simulink model "active_vehicle_ESP_Control"  (R2020a)
settings: Solver=ode4  StartTime=0.0  StopTime=inf  FixedStep=1e-3  RelTol=1e-3
InitFcn:
  | clear mex
model workspace (MAT data in the model file):
  inChnlList : object (value not decoded)
  inChnlListInternal : object (value not decoded)
  outChnlList : object (value not decoded)
  outChnlListInternal : object (value not decoded)
undefined symbols (not defined in the file or in its folder): DiscIntNeverNeededParam, vicrt_initcallback, vicrt_initmexcallback, vicrt_inputfile, vicrt_simulationmanager
libraries: simulink x1
(part 6 of 6)

== system active_vehicle_ESP_Control/Vehicle/VI-CarRealTime/Input_Bus/Inputs/Irregularity/road ==
  BCroad : BusCreator  Inputs=4
  L1_def_val : Constant  Value=0
  L2_def_val : Constant  Value=0
  R1_def_val : Constant  Value=0
  R2_def_val : Constant  Value=0
  road : Outport
  wires:
  BCroad/1 -> road/1  "road"
  L1_def_val/1 -> BCroad/1  "L1"
  L2_def_val/1 -> BCroad/2  "L2"
  R1_def_val/1 -> BCroad/3  "R1"
  R2_def_val/1 -> BCroad/4  "R2"

== system active_vehicle_ESP_Control/Vehicle/VI-CarRealTime/Input_Bus/Inputs/Main_Bumpstop/activity_flag ==
  BCactivity_flag : BusCreator  Inputs=4
  L1_def_val : Constant
  L2_def_val : Constant
  R1_def_val : Constant
  R2_def_val : Constant
  activity_flag : Outport
  wires:
  BCactivity_flag/1 -> activity_flag/1  "activity_flag"
  L1_def_val/1 -> BCactivity_flag/1  "L1"
  L2_def_val/1 -> BCactivity_flag/2  "L2"
  R1_def_val/1 -> BCactivity_flag/3  "R1"
  R2_def_val/1 -> BCactivity_flag/4  "R2"

== system active_vehicle_ESP_Control/Vehicle/VI-CarRealTime/Input_Bus/Inputs/Main_Bumpstop/force ==
  BCforce : BusCreator  Inputs=4
  L1_def_val : Constant  Value=0
  L2_def_val : Constant  Value=0
  R1_def_val : Constant  Value=0
  R2_def_val : Constant  Value=0
  force : Outport
  wires:
  BCforce/1 -> force/1  "force"
  L1_def_val/1 -> BCforce/1  "L1"
  L2_def_val/1 -> BCforce/2  "L2"
  R1_def_val/1 -> BCforce/3  "R1"
  R2_def_val/1 -> BCforce/4  "R2"

== system active_vehicle_ESP_Control/Vehicle/VI-CarRealTime/Input_Bus/Inputs/Main_Damper/activity_flag ==
  BCactivity_flag : BusCreator  Inputs=4
  L1_def_val : Constant
  L2_def_val : Constant
  R1_def_val : Constant
  R2_def_val : Constant
  activity_flag : Outport
  wires:
  BCactivity_flag/1 -> activity_flag/1  "activity_flag"
  L1_def_val/1 -> BCactivity_flag/1  "L1"
  L2_def_val/1 -> BCactivity_flag/2  "L2"
  R1_def_val/1 -> BCactivity_flag/3  "R1"
  R2_def_val/1 -> BCactivity_flag/4  "R2"

== system active_vehicle_ESP_Control/Vehicle/VI-CarRealTime/Input_Bus/Inputs/Main_Damper/force ==
  BCforce : BusCreator  Inputs=4
  L1_def_val : Constant  Value=0
  L2_def_val : Constant  Value=0
  R1_def_val : Constant  Value=0
  R2_def_val : Constant  Value=0
  force : Outport
  wires:
  BCforce/1 -> force/1  "force"
  L1_def_val/1 -> BCforce/1  "L1"
  L2_def_val/1 -> BCforce/2  "L2"
  R1_def_val/1 -> BCforce/3  "R1"
  R2_def_val/1 -> BCforce/4  "R2"

== system active_vehicle_ESP_Control/Vehicle/VI-CarRealTime/Input_Bus/Inputs/Main_Inerter/activity_flag ==
  BCactivity_flag : BusCreator  Inputs=4
  L1_def_val : Constant
  L2_def_val : Constant
  R1_def_val : Constant
  R2_def_val : Constant
  activity_flag : Outport
  wires:
  BCactivity_flag/1 -> activity_flag/1  "activity_flag"
  L1_def_val/1 -> BCactivity_flag/1  "L1"
  L2_def_val/1 -> BCactivity_flag/2  "L2"
  R1_def_val/1 -> BCactivity_flag/3  "R1"
  R2_def_val/1 -> BCactivity_flag/4  "R2"

== system active_vehicle_ESP_Control/Vehicle/VI-CarRealTime/Input_Bus/Inputs/Main_Inerter/force ==
  BCforce : BusCreator  Inputs=4
  L1_def_val : Constant  Value=0
  L2_def_val : Constant  Value=0
  R1_def_val : Constant  Value=0
  R2_def_val : Constant  Value=0
  force : Outport
  wires:
  BCforce/1 -> force/1  "force"
  L1_def_val/1 -> BCforce/1  "L1"
  L2_def_val/1 -> BCforce/2  "L2"
  R1_def_val/1 -> BCforce/3  "R1"
  R2_def_val/1 -> BCforce/4  "R2"

== system active_vehicle_ESP_Control/Vehicle/VI-CarRealTime/Input_Bus/Inputs/Main_Reboundstop/activity_flag ==
  BCactivity_flag : BusCreator  Inputs=4
  L1_def_val : Constant
  L2_def_val : Constant
  R1_def_val : Constant
  R2_def_val : Constant
  activity_flag : Outport
  wires:
  BCactivity_flag/1 -> activity_flag/1  "activity_flag"
  L1_def_val/1 -> BCactivity_flag/1  "L1"
  L2_def_val/1 -> BCactivity_flag/2  "L2"
  R1_def_val/1 -> BCactivity_flag/3  "R1"
  R2_def_val/1 -> BCactivity_flag/4  "R2"

== system active_vehicle_ESP_Control/Vehicle/VI-CarRealTime/Input_Bus/Inputs/Main_Reboundstop/force ==
  BCforce : BusCreator  Inputs=4
  L1_def_val : Constant  Value=0
  L2_def_val : Constant  Value=0
  R1_def_val : Constant  Value=0
  R2_def_val : Constant  Value=0
  force : Outport
  wires:
  BCforce/1 -> force/1  "force"
  L1_def_val/1 -> BCforce/1  "L1"
  L2_def_val/1 -> BCforce/2  "L2"
  R1_def_val/1 -> BCforce/3  "R1"
  R2_def_val/1 -> BCforce/4  "R2"

== system active_vehicle_ESP_Control/Vehicle/VI-CarRealTime/Input_Bus/Inputs/Main_Spring/activity_flag ==
  BCactivity_flag : BusCreator  Inputs=4
  L1_def_val : Constant
  L2_def_val : Constant
  R1_def_val : Constant
  R2_def_val : Constant
  activity_flag : Outport
  wires:
  BCactivity_flag/1 -> activity_flag/1  "activity_flag"
  L1_def_val/1 -> BCactivity_flag/1  "L1"
  L2_def_val/1 -> BCactivity_flag/2  "L2"
  R1_def_val/1 -> BCactivity_flag/3  "R1"
  R2_def_val/1 -> BCactivity_flag/4  "R2"

== system active_vehicle_ESP_Control/Vehicle/VI-CarRealTime/Input_Bus/Inputs/Main_Spring/force ==
  BCforce : BusCreator  Inputs=4
  L1_def_val : Constant  Value=0
  L2_def_val : Constant  Value=0
  R1_def_val : Constant  Value=0
  R2_def_val : Constant  Value=0
  force : Outport
  wires:
  BCforce/1 -> force/1  "force"
  L1_def_val/1 -> BCforce/1  "L1"
  L2_def_val/1 -> BCforce/2  "L2"
  R1_def_val/1 -> BCforce/3  "R1"
  R2_def_val/1 -> BCforce/4  "R2"

== system active_vehicle_ESP_Control/Vehicle/VI-CarRealTime/Input_Bus/Inputs/Mono_Element/Bumpstop_Damper ==
  BCBumpstop_Damper : BusCreator  Inputs=2
  front_def_val : Constant  Value=0
  rear_def_val : Constant  Value=0
  Bumpstop_Damper : Outport
  wires:
  BCBumpstop_Damper/1 -> Bumpstop_Damper/1  "Bumpstop_Damper"
  front_def_val/1 -> BCBumpstop_Damper/1  "front"
  rear_def_val/1 -> BCBumpstop_Damper/2  "rear"

== system active_vehicle_ESP_Control/Vehicle/VI-CarRealTime/Input_Bus/Inputs/Mono_Element/Bumpstop_Damper_activity_flag ==
  BCBumpstop_Damper_activity_flag : BusCreator  Inputs=2
  front_def_val : Constant
  rear_def_val : Constant
  Bumpstop_Damper_activity_flag : Outport
  wires:
  BCBumpstop_Damper_activity_flag/1 -> Bumpstop_Damper_activity_flag/1  "Bumpstop_Damper_activity_flag"
  front_def_val/1 -> BCBumpstop_Damper_activity_flag/1  "front"
  rear_def_val/1 -> BCBumpstop_Damper_activity_flag/2  "rear"

== system active_vehicle_ESP_Control/Vehicle/VI-CarRealTime/Input_Bus/Inputs/Mono_Element/Bumpstop_Spring ==
  BCBumpstop_Spring : BusCreator  Inputs=2
  front_def_val : Constant  Value=0
  rear_def_val : Constant  Value=0
  Bumpstop_Spring : Outport
  wires:
  BCBumpstop_Spring/1 -> Bumpstop_Spring/1  "Bumpstop_Spring"
  front_def_val/1 -> BCBumpstop_Spring/1  "front"
  rear_def_val/1 -> BCBumpstop_Spring/2  "rear"

== system active_vehicle_ESP_Control/Vehicle/VI-CarRealTime/Input_Bus/Inputs/Mono_Element/Bumpstop_Spring_activity_flag ==
  BCBumpstop_Spring_activity_flag : BusCreator  Inputs=2
  front_def_val : Constant
  rear_def_val : Constant
  Bumpstop_Spring_activity_flag : Outport
  wires:
  BCBumpstop_Spring_activity_flag/1 -> Bumpstop_Spring_activity_flag/1  "Bumpstop_Spring_activity_flag"
  front_def_val/1 -> BCBumpstop_Spring_activity_flag/1  "front"
  rear_def_val/1 -> BCBumpstop_Spring_activity_flag/2  "rear"

== system active_vehicle_ESP_Control/Vehicle/VI-CarRealTime/Input_Bus/Inputs/Mono_Element/Damper ==
  BCDamper : BusCreator  Inputs=2
  front_def_val : Constant  Value=0
  rear_def_val : Constant  Value=0
  Damper : Outport
  wires:
  BCDamper/1 -> Damper/1  "Damper"
  front_def_val/1 -> BCDamper/1  "front"
  rear_def_val/1 -> BCDamper/2  "rear"

== system active_vehicle_ESP_Control/Vehicle/VI-CarRealTime/Input_Bus/Inputs/Mono_Element/Damper_activity_flag ==
  BCDamper_activity_flag : BusCreator  Inputs=2
  front_def_val : Constant
  rear_def_val : Constant
  Damper_activity_flag : Outport
  wires:
  BCDamper_activity_flag/1 -> Damper_activity_flag/1  "Damper_activity_flag"
  front_def_val/1 -> BCDamper_activity_flag/1  "front"
  rear_def_val/1 -> BCDamper_activity_flag/2  "rear"

== system active_vehicle_ESP_Control/Vehicle/VI-CarRealTime/Input_Bus/Inputs/Mono_Element/Inerter ==
  BCInerter : BusCreator  Inputs=2
  front_def_val : Constant  Value=0
  rear_def_val : Constant  Value=0
  Inerter : Outport
  wires:
  BCInerter/1 -> Inerter/1  "Inerter"
  front_def_val/1 -> BCInerter/1  "front"
  rear_def_val/1 -> BCInerter/2  "rear"

== system active_vehicle_ESP_Control/Vehicle/VI-CarRealTime/Input_Bus/Inputs/Mono_Element/Inerter_activity_flag ==
  BCInerter_activity_flag : BusCreator  Inputs=2
  front_def_val : Constant
  rear_def_val : Constant
  Inerter_activity_flag : Outport
  wires:
  BCInerter_activity_flag/1 -> Inerter_activity_flag/1  "Inerter_activity_flag"
  front_def_val/1 -> BCInerter_activity_flag/1  "front"
  rear_def_val/1 -> BCInerter_activity_flag/2  "rear"

== system active_vehicle_ESP_Control/Vehicle/VI-CarRealTime/Input_Bus/Inputs/Mono_Element/Reboundstop_Damper ==
  BCReboundstop_Damper : BusCreator  Inputs=2
  front_def_val : Constant  Value=0
  rear_def_val : Constant  Value=0
  Reboundstop_Damper : Outport
  wires:
  BCReboundstop_Damper/1 -> Reboundstop_Damper/1  "Reboundstop_Damper"
  front_def_val/1 -> BCReboundstop_Damper/1  "front"
  rear_def_val/1 -> BCReboundstop_Damper/2  "rear"

== system active_vehicle_ESP_Control/Vehicle/VI-CarRealTime/Input_Bus/Inputs/Mono_Element/Reboundstop_Damper_activity_flag ==
  BCReboundstop_Damper_activity_flag : BusCreator  Inputs=2
  front_def_val : Constant
  rear_def_val : Constant
  Reboundstop_Damper_activity_flag : Outport
  wires:
  BCReboundstop_Damper_activity_flag/1 -> Reboundstop_Damper_activity_flag/1  "Reboundstop_Damper_activity_flag"
  front_def_val/1 -> BCReboundstop_Damper_activity_flag/1  "front"
  rear_def_val/1 -> BCReboundstop_Damper_activity_flag/2  "rear"

== system active_vehicle_ESP_Control/Vehicle/VI-CarRealTime/Input_Bus/Inputs/Mono_Element/Reboundstop_Spring ==
  BCReboundstop_Spring : BusCreator  Inputs=2
  front_def_val : Constant  Value=0
  rear_def_val : Constant  Value=0
  Reboundstop_Spring : Outport
  wires:
  BCReboundstop_Spring/1 -> Reboundstop_Spring/1  "Reboundstop_Spring"
  front_def_val/1 -> BCReboundstop_Spring/1  "front"
  rear_def_val/1 -> BCReboundstop_Spring/2  "rear"

== system active_vehicle_ESP_Control/Vehicle/VI-CarRealTime/Input_Bus/Inputs/Mono_Element/Reboundstop_Spring_activity_flag ==
  BCReboundstop_Spring_activity_flag : BusCreator  Inputs=2
  front_def_val : Constant
  rear_def_val : Constant
  Reboundstop_Spring_activity_flag : Outport
  wires:
  BCReboundstop_Spring_activity_flag/1 -> Reboundstop_Spring_activity_flag/1  "Reboundstop_Spring_activity_flag"
  front_def_val/1 -> BCReboundstop_Spring_activity_flag/1  "front"
  rear_def_val/1 -> BCReboundstop_Spring_activity_flag/2  "rear"

== system active_vehicle_ESP_Control/Vehicle/VI-CarRealTime/Input_Bus/Inputs/Mono_Element/Roll_Damper ==
  BCRoll_Damper : BusCreator  Inputs=2
  front_def_val : Constant  Value=0
  rear_def_val : Constant  Value=0
  Roll_Damper : Outport
  wires:
  BCRoll_Damper/1 -> Roll_Damper/1  "Roll_Damper"
  front_def_val/1 -> BCRoll_Damper/1  "front"
  rear_def_val/1 -> BCRoll_Damper/2  "rear"

== system active_vehicle_ESP_Control/Vehicle/VI-CarRealTime/Input_Bus/Inputs/Mono_Element/Roll_Damper_activity_flag ==
  BCRoll_Damper_activity_flag : BusCreator  Inputs=2
  front_def_val : Constant
  rear_def_val : Constant
  Roll_Damper_activity_flag : Outport
  wires:
  BCRoll_Damper_activity_flag/1 -> Roll_Damper_activity_flag/1  "Roll_Damper_activity_flag"
  front_def_val/1 -> BCRoll_Damper_activity_flag/1  "front"
  rear_def_val/1 -> BCRoll_Damper_activity_flag/2  "rear"

== system active_vehicle_ESP_Control/Vehicle/VI-CarRealTime/Input_Bus/Inputs/Mono_Element/Spring ==
  BCSpring : BusCreator  Inputs=2
  front_def_val : Constant  Value=0
  rear_def_val : Constant  Value=0
  Spring : Outport
  wires:
  BCSpring/1 -> Spring/1  "Spring"
  front_def_val/1 -> BCSpring/1  "front"
  rear_def_val/1 -> BCSpring/2  "rear"

== system active_vehicle_ESP_Control/Vehicle/VI-CarRealTime/Input_Bus/Inputs/Mono_Element/Spring_activity_flag ==
  BCSpring_activity_flag : BusCreator  Inputs=2
  front_def_val : Constant
  rear_def_val : Constant
  Spring_activity_flag : Outport
  wires:
  BCSpring_activity_flag/1 -> Spring_activity_flag/1  "Spring_activity_flag"
  front_def_val/1 -> BCSpring_activity_flag/1  "front"
  rear_def_val/1 -> BCSpring_activity_flag/2  "rear"

== system active_vehicle_ESP_Control/Vehicle/VI-CarRealTime/Input_Bus/Inputs/Rear_Steering_Actuator_disp/str_swa ==
  BCstr_swa : BusCreator  Inputs=2
  left_def_val : Constant  Value=0
  right_def_val : Constant  Value=0
  str_swa : Outport
  wires:
  BCstr_swa/1 -> str_swa/1  "str_swa"
  left_def_val/1 -> BCstr_swa/1  "left"
  right_def_val/1 -> BCstr_swa/2  "right"

== system active_vehicle_ESP_Control/Vehicle/VI-CarRealTime/Input_Bus/Inputs/Steering/steer_at_spindle ==
  BCsteer_at_spindle : BusCreator  Inputs=4
  L1_def_val : Constant  Value=0
  L2_def_val : Constant  Value=0
  R1_def_val : Constant  Value=0
  R2_def_val : Constant  Value=0
  steer_at_spindle : Outport
  wires:
  BCsteer_at_spindle/1 -> steer_at_spindle/1  "steer_at_spindle"
  L1_def_val/1 -> BCsteer_at_spindle/1  "L1"
  L2_def_val/1 -> BCsteer_at_spindle/2  "L2"
  R1_def_val/1 -> BCsteer_at_spindle/3  "R1"
  R2_def_val/1 -> BCsteer_at_spindle/4  "R2"

== system active_vehicle_ESP_Control/Vehicle/VI-CarRealTime/Input_Bus/Inputs/Subsystem_Activation/Internal_Brake_System_Activity ==
  BCInternal_Brake_System_Activity : BusCreator  Inputs=4
  L1_def_val : Constant
  L2_def_val : Constant
  R1_def_val : Constant
  R2_def_val : Constant
  Internal_Brake_System_Activity : Outport
  wires:
  BCInternal_Brake_System_Activity/1 -> Internal_Brake_System_Activity/1  "Internal_Brake_System_Activity"
  L1_def_val/1 -> BCInternal_Brake_System_Activity/1  "L1"
  L2_def_val/1 -> BCInternal_Brake_System_Activity/2  "L2"
  R1_def_val/1 -> BCInternal_Brake_System_Activity/3  "R1"
  R2_def_val/1 -> BCInternal_Brake_System_Activity/4  "R2"

== system active_vehicle_ESP_Control/Vehicle/VI-CarRealTime/Input_Bus/Inputs/Subsystem_Activation/Tire_Force_x ==
  BCTire_Force_x : BusCreator  Inputs=4
  L1_def_val : Constant
  L2_def_val : Constant
  R1_def_val : Constant
  R2_def_val : Constant
  Tire_Force_x : Outport
  wires:
  BCTire_Force_x/1 -> Tire_Force_x/1  "Tire_Force_x"
  L1_def_val/1 -> BCTire_Force_x/1  "L1"
  L2_def_val/1 -> BCTire_Force_x/2  "L2"
  R1_def_val/1 -> BCTire_Force_x/3  "R1"
  R2_def_val/1 -> BCTire_Force_x/4  "R2"

== system active_vehicle_ESP_Control/Vehicle/VI-CarRealTime/Input_Bus/Inputs/Subsystem_Activation/Tire_Force_y ==
  BCTire_Force_y : BusCreator  Inputs=4
  L1_def_val : Constant
  L2_def_val : Constant
  R1_def_val : Constant
  R2_def_val : Constant
  Tire_Force_y : Outport
  wires:
  BCTire_Force_y/1 -> Tire_Force_y/1  "Tire_Force_y"
  L1_def_val/1 -> BCTire_Force_y/1  "L1"
  L2_def_val/1 -> BCTire_Force_y/2  "L2"
  R1_def_val/1 -> BCTire_Force_y/3  "R1"
  R2_def_val/1 -> BCTire_Force_y/4  "R2"

== system active_vehicle_ESP_Control/Vehicle/VI-CarRealTime/Input_Bus/Inputs/Subsystem_Activation/Tire_Force_z ==
  BCTire_Force_z : BusCreator  Inputs=4
  L1_def_val : Constant
  L2_def_val : Constant
  R1_def_val : Constant
  R2_def_val : Constant
  Tire_Force_z : Outport
  wires:
  BCTire_Force_z/1 -> Tire_Force_z/1  "Tire_Force_z"
  L1_def_val/1 -> BCTire_Force_z/1  "L1"
  L2_def_val/1 -> BCTire_Force_z/2  "L2"
  R1_def_val/1 -> BCTire_Force_z/3  "R1"
  R2_def_val/1 -> BCTire_Force_z/4  "R2"

== system active_vehicle_ESP_Control/Vehicle/VI-CarRealTime/Input_Bus/Inputs/Subsystem_Activation/Tire_Moment_x ==
  BCTire_Moment_x : BusCreator  Inputs=4
  L1_def_val : Constant
  L2_def_val : Constant
  R1_def_val : Constant
  R2_def_val : Constant
  Tire_Moment_x : Outport
  wires:
  BCTire_Moment_x/1 -> Tire_Moment_x/1  "Tire_Moment_x"
  L1_def_val/1 -> BCTire_Moment_x/1  "L1"
  L2_def_val/1 -> BCTire_Moment_x/2  "L2"
  R1_def_val/1 -> BCTire_Moment_x/3  "R1"
  R2_def_val/1 -> BCTire_Moment_x/4  "R2"

== system active_vehicle_ESP_Control/Vehicle/VI-CarRealTime/Input_Bus/Inputs/Subsystem_Activation/Tire_Moment_y ==
  BCTire_Moment_y : BusCreator  Inputs=4
  L1_def_val : Constant
  L2_def_val : Constant
  R1_def_val : Constant
  R2_def_val : Constant
  Tire_Moment_y : Outport
  wires:
  BCTire_Moment_y/1 -> Tire_Moment_y/1  "Tire_Moment_y"
  L1_def_val/1 -> BCTire_Moment_y/1  "L1"
  L2_def_val/1 -> BCTire_Moment_y/2  "L2"
  R1_def_val/1 -> BCTire_Moment_y/3  "R1"
  R2_def_val/1 -> BCTire_Moment_y/4  "R2"

== system active_vehicle_ESP_Control/Vehicle/VI-CarRealTime/Input_Bus/Inputs/Subsystem_Activation/Tire_Moment_z ==
  BCTire_Moment_z : BusCreator  Inputs=4
  L1_def_val : Constant
  L2_def_val : Constant
  R1_def_val : Constant
  R2_def_val : Constant
  Tire_Moment_z : Outport
  wires:
  BCTire_Moment_z/1 -> Tire_Moment_z/1  "Tire_Moment_z"
  L1_def_val/1 -> BCTire_Moment_z/1  "L1"
  L2_def_val/1 -> BCTire_Moment_z/2  "L2"
  R1_def_val/1 -> BCTire_Moment_z/3  "R1"
  R2_def_val/1 -> BCTire_Moment_z/4  "R2"

== system active_vehicle_ESP_Control/Vehicle/VI-CarRealTime/Input_Bus/Inputs/Third_Element/Damper_activity_flag ==
  BCDamper_activity_flag : BusCreator  Inputs=2
  front_def_val : Constant
  rear_def_val : Constant
  Damper_activity_flag : Outport
  wires:
  BCDamper_activity_flag/1 -> Damper_activity_flag/1  "Damper_activity_flag"
  front_def_val/1 -> BCDamper_activity_flag/1  "front"
  rear_def_val/1 -> BCDamper_activity_flag/2  "rear"

== system active_vehicle_ESP_Control/Vehicle/VI-CarRealTime/Input_Bus/Inputs/Third_Element/Damper_force ==
  BCDamper_force : BusCreator  Inputs=2
  front_def_val : Constant  Value=0
  rear_def_val : Constant  Value=0
  Damper_force : Outport
  wires:
  BCDamper_force/1 -> Damper_force/1  "Damper_force"
  front_def_val/1 -> BCDamper_force/1  "front"
  rear_def_val/1 -> BCDamper_force/2  "rear"

== system active_vehicle_ESP_Control/Vehicle/VI-CarRealTime/Input_Bus/Inputs/Third_Element/Spring ==
  BCSpring : BusCreator  Inputs=2
  front_def_val : Constant  Value=0
  rear_def_val : Constant  Value=0
  Spring : Outport
  wires:
  BCSpring/1 -> Spring/1  "Spring"
  front_def_val/1 -> BCSpring/1  "front"
  rear_def_val/1 -> BCSpring/2  "rear"

== system active_vehicle_ESP_Control/Vehicle/VI-CarRealTime/Input_Bus/Inputs/Third_Element/Spring_activity_flag ==
  BCSpring_activity_flag : BusCreator  Inputs=2
  front_def_val : Constant
  rear_def_val : Constant
  Spring_activity_flag : Outport
  wires:
  BCSpring_activity_flag/1 -> Spring_activity_flag/1  "Spring_activity_flag"
  front_def_val/1 -> BCSpring_activity_flag/1  "front"
  rear_def_val/1 -> BCSpring_activity_flag/2  "rear"

== system active_vehicle_ESP_Control/Vehicle/VI-CarRealTime/Input_Bus/Inputs/Tire_Force/Fx ==
  BCFx : BusCreator  Inputs=4
  L1_def_val : Constant  Value=0
  L2_def_val : Constant  Value=0
  R1_def_val : Constant  Value=0
  R2_def_val : Constant  Value=0
  Fx : Outport
  wires:
  BCFx/1 -> Fx/1  "Fx"
  L1_def_val/1 -> BCFx/1  "L1"
  L2_def_val/1 -> BCFx/2  "L2"
  R1_def_val/1 -> BCFx/3  "R1"
  R2_def_val/1 -> BCFx/4  "R2"

== system active_vehicle_ESP_Control/Vehicle/VI-CarRealTime/Input_Bus/Inputs/Tire_Force/Fy ==
  BCFy : BusCreator  Inputs=4
  L1_def_val : Constant  Value=0
  L2_def_val : Constant  Value=0
  R1_def_val : Constant  Value=0
  R2_def_val : Constant  Value=0
  Fy : Outport
  wires:
  BCFy/1 -> Fy/1  "Fy"
  L1_def_val/1 -> BCFy/1  "L1"
  L2_def_val/1 -> BCFy/2  "L2"
  R1_def_val/1 -> BCFy/3  "R1"
  R2_def_val/1 -> BCFy/4  "R2"

== system active_vehicle_ESP_Control/Vehicle/VI-CarRealTime/Input_Bus/Inputs/Tire_Force/Fz ==
  BCFz : BusCreator  Inputs=4
  L1_def_val : Constant  Value=0
  L2_def_val : Constant  Value=0
  R1_def_val : Constant  Value=0
  R2_def_val : Constant  Value=0
  Fz : Outport
  wires:
  BCFz/1 -> Fz/1  "Fz"
  L1_def_val/1 -> BCFz/1  "L1"
  L2_def_val/1 -> BCFz/2  "L2"
  R1_def_val/1 -> BCFz/3  "R1"
  R2_def_val/1 -> BCFz/4  "R2"

== system active_vehicle_ESP_Control/Vehicle/VI-CarRealTime/Input_Bus/Inputs/Tire_Moment/Mx ==
  BCMx : BusCreator  Inputs=4
  L1_def_val : Constant  Value=0
  L2_def_val : Constant  Value=0
  R1_def_val : Constant  Value=0
  R2_def_val : Constant  Value=0
  Mx : Outport
  wires:
  BCMx/1 -> Mx/1  "Mx"
  L1_def_val/1 -> BCMx/1  "L1"
  L2_def_val/1 -> BCMx/2  "L2"
  R1_def_val/1 -> BCMx/3  "R1"
  R2_def_val/1 -> BCMx/4  "R2"

== system active_vehicle_ESP_Control/Vehicle/VI-CarRealTime/Input_Bus/Inputs/Tire_Moment/My ==
  BCMy : BusCreator  Inputs=4
  L1_def_val : Constant  Value=0
  L2_def_val : Constant  Value=0
  R1_def_val : Constant  Value=0
  R2_def_val : Constant  Value=0
  My : Outport
  wires:
  BCMy/1 -> My/1  "My"
  L1_def_val/1 -> BCMy/1  "L1"
  L2_def_val/1 -> BCMy/2  "L2"
  R1_def_val/1 -> BCMy/3  "R1"
  R2_def_val/1 -> BCMy/4  "R2"

== system active_vehicle_ESP_Control/Vehicle/VI-CarRealTime/Input_Bus/Inputs/Tire_Moment/Mz ==
  BCMz : BusCreator  Inputs=4
  L1_def_val : Constant  Value=0
  L2_def_val : Constant  Value=0
  R1_def_val : Constant  Value=0
  R2_def_val : Constant  Value=0
  Mz : Outport
  wires:
  BCMz/1 -> Mz/1  "Mz"
  L1_def_val/1 -> BCMz/1  "L1"
  L2_def_val/1 -> BCMz/2  "L2"
  R1_def_val/1 -> BCMz/3  "R1"
  R2_def_val/1 -> BCMz/4  "R2"

== system active_vehicle_ESP_Control/Vehicle/VI-CarRealTime/Input_Bus/Inputs/Wheel_driving/moment ==
  BCmoment : BusCreator  Inputs=4
  L1_def_val : Constant  Value=0
  L2_def_val : Constant  Value=0
  R1_def_val : Constant  Value=0
  R2_def_val : Constant  Value=0
  moment : Outport
  wires:
  BCmoment/1 -> moment/1  "moment"
  L1_def_val/1 -> BCmoment/1  "L1"
  L2_def_val/1 -> BCmoment/2  "L2"
  R1_def_val/1 -> BCmoment/3  "R1"
  R2_def_val/1 -> BCmoment/4  "R2"

== matlab function active_vehicle_ESP_Control/Driveline/Clutch/Embedded MATLAB Function ==
  data: x input; clh output; x1 input; x2 input
function clh =clutch_activity_step(x,x1,x2)
y1=0;
y2=1;
n=length(x);
clh=zeros(n,1);
if (x2 < x1)
    tmp=x2;
    x2=x1;
    x1=tmp;
    tmp=y2;
    y2=y1;
    y1=tmp;
end
for i=1:n
    if x(i)<=x1
        clh(i)=y1;
    elseif x(i)>x2
        clh(i)=y2;
    else
        a = y2-y1;
        delta =(x(i)-x1)/(x2-x1);
        clh(i)=(y1+a*delta^2*(3.0-2.0*delta));
    end
end

== matlab function active_vehicle_ESP_Control/ESP/ESP/Embedded MATLAB Function ==
  data: SideSlip input; FL output; FR output; RL output; RR output; yawr input; SWA input; Vx input; overSteerRate output; throttleOffTrigger output; yawrT output; WheelBase input; steerRatio input
function [FL,FR, RL, RR,overSteerRate, throttleOffTrigger,yawrT] = fcn(SideSlip,yawr,SWA,Vx, WheelBase,steerRatio) 
%ESP controller, control target: (yaw rate desired)-(yaw rate actual)
% Vehicle parameters
p=WheelBase; % WheelBase
yawrT=Vx/3.6*tan(SWA*steerRatio)/p; % Desired Yaw Rate
YawRThreshold=0.0051; % Yaw Rate threshold [rad/sec](ESP OFF)
YawRErrorThreshold=1.5; % Yaw Rate Error threshold [rad/sec](Throttle OFF)
%
FL=0;
FR=0;
RL=0;
RR=0;
throttleOffTrigger = 0.0;
yawrError = yawrT-yawr;
overSteerRate = - yawrError * sign(yawr);
if (yawr>0)  %left turn
    if (yawrError)<-YawRThreshold %%oversteering
            RL=abs(yawrError);
            FR=abs(yawrError);
            %throttleOffTrigger = 1.0;        
    end;            
    if (yawrError)>YawRThreshold %%understeering
           FL=abs(yawrError);
           RR=abs(yawrError);
           if abs(yawrError)>YawRErrorThreshold
               throttleOffTrigger = 1.0;
           end
    end;         
end;
if (yawr<0) % right turn
    if (yawrError)>YawRThreshold %%oversteering
            RR=abs(yawrError);
            FL=abs(yawrError);
            %throttleOffTrigger = 1.0;
    end;            
    if (yawrError)<-YawRThreshold %%understeering
            FR=abs(yawrError);
            RL=abs(yawrError); 
            if abs(yawrError)>YawRErrorThreshold
                throttleOffTrigger = 1.0;
            end         
    end;        
end;

== matlab function active_vehicle_ESP_Control/Driveline/Clutch/Embedded MATLAB Function1 ==
  data: x input; clh output; x1 input; x2 input
function clh =clutch_activity_step(x,x1,x2)
y1=0;
y2=1;
n=length(x);
clh=zeros(n,1);
if (x2 < x1)
    tmp=x2;
    x2=x1;
    x1=tmp;
    tmp=y2;
    y2=y1;
    y1=tmp;
end
for i=1:n
    if x(i)<=x1
        clh(i)=y1;
    elseif x(i)>x2
        clh(i)=y2;
    else
        a = y2-y1;
        delta =(x(i)-x1)/(x2-x1);
        clh(i)=y1+a*delta^2*(3.0-2.0*delta);
    end
end

== matlab function active_vehicle_ESP_Control/Driveline/Engine/Engine Maps/Rpm control/Embedded MATLAB Function ==
  data: x input; thr output; x1 input; x2 input
function thr =thr_step(x,x1,x2)
y1=1;
y2=0;
n=length(x);
thr=zeros(n,1);
if (x2 < x1)
    tmp=x2;
    x2=x1;
    x1=tmp;
    tmp=y2;
    y2=y1;
    y1=tmp;
end
for i=1:n
    if x(i)<=x1
        thr(i)=y1;
    elseif x(i)>x2
        thr(i)=y2;
    else
        a = y2-y1;
        delta =(x(i)-x1)/(x2-x1);
        thr(i)=y1+a*delta^2*(3.0-2.0*delta);
    end
end
